simulink model "devCreateSdat"  (R2018b)
settings: Solver=VariableStepDiscrete  StartTime=0  StopTime=1  MaxStep=1  RelTol=1e-3  EnableMultiTasking=on
InitFcn:
  | load('DE_TRY2010_13_averageYear')
libraries: carnot x1, CreateSdat x1
settings Model: Creator=drhf  LastModifiedBy=drhf
settings DataIOCC: SaveFormat=Array  SignalLoggingSaveFormat=ModelDataLogs
settings OptimizationCC: ExpressionDepthLimit=2147483647  LifeSpan=inf
settings DebuggingCC: UnderspecifiedInitializationDetection=Classic  MergeDetectMultiDrivingBlocksExec=none  SolverPrmCheckMsg=warning  FcnCallInpInsideContextMsg=warning  StateNameClashWarn=warning  SFUnexpectedBacktrackingDiag=warning  SFNoUnconditionalDefaultTransitionDiag=warning  SFExecutionAtInitializationDiag=none
settings HardwareCC: ProdBitPerPointer=32  ProdBitPerSizeT=32  ProdBitPerPtrDiffT=32  ProdLargestAtomicFloat=None  ProdIntDivRoundTo=Undefined  ProdEndianess=Unspecified  ProdWordSize=32  ProdHWDeviceType=32-bit Generic
settings ModelReferenceCC: PropagateSignalLabelsOutOfModel=off
settings SFSimCC: SimUseLocalCustomCode=off
settings RTWCC: RTWUseLocalCustomCode=off
settings CodeAppCC: StateflowObjectComments=on
settings GRTTargetCC: TargetLangStandard=C89/C90 (ANSI)  GeneratePreprocessorConditionals=Disable all  CombineOutputUpdateFcns=off  GRTInterface=on
settings ConfigComp: CovMetricSettings=dw  CovHtmlReporting=on  CovSaveCumulativeToWorkspaceVar=on  CovSaveSingleToWorkspaceVar=on  CovExternalEMLEnable=off

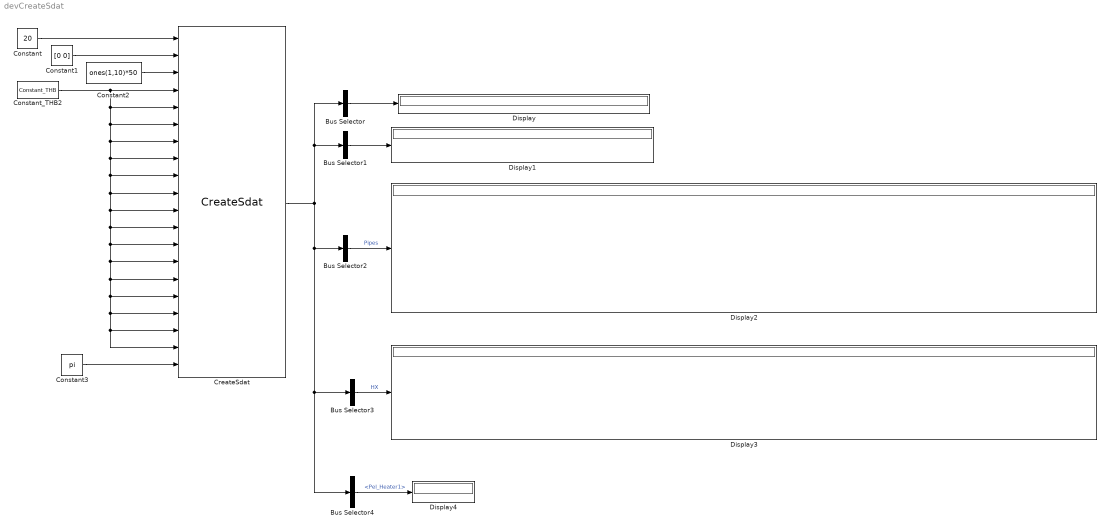
== system devCreateSdat ==
  Bus Selector : BusSelector  OutputSignals=Tamb,energy,volume,storageType  OutputAsBus=on
  Bus Selector1 : BusSelector  OutputSignals=Tnodes  OutputAsBus=on
  Bus Selector2 : BusSelector  OutputSignals=THBin_pipe1,THBout_pipe1,THBin_pipe2,THBout_pipe2,THBin_pipe3,THBout_pipe3,THBin_pipe4,THBout_pipe4,THBin_pipe5,THBout_pipe5  OutputAsBus=on
  Bus Selector3 : BusSelector  OutputSignals=THBin_hx1,THBout_hx1,THBin_hx2,THBout_hx2,THBin_hx3,THBout_hx3  OutputAsBus=on
  Bus Selector4 : BusSelector  OutputSignals=Pel_Heater1
  Constant : Constant  Value=20
  Constant1 : Constant  Value=[0 0]
  Constant2 : Constant  Value=ones(1,10)*50
  Constant3 : Constant  Value=pi
  Constant_THB2 : carnot/Source/Simple/Constant_THB  t=30  mdot=0  p=1e5  mID=No Pressure Drop  fluid=Water  mix=0  mix2=0  mix3=0  dia=0.02  hgt=0
      settings: SourceProductName=Carnot
  CreateSdat : CreateSdat/CreateSdat  volume=0.5  stgtype=1
  Display{,1..4} (5 alike) : Display
  wires:
  CreateSdat/1 -> Bus Selector2/1, Bus Selector3/1, Bus Selector4/1, Bus Selector1/1, Bus Selector/1
  Constant_THB2/1 -> CreateSdat/11, CreateSdat/13, CreateSdat/14, CreateSdat/15, CreateSdat/16, CreateSdat/17, CreateSdat/18, CreateSdat/19, CreateSdat/12, CreateSdat/10, CreateSdat/9, CreateSdat/8, CreateSdat/7, CreateSdat/6, CreateSdat/5, CreateSdat/4
  Constant/1 -> CreateSdat/1
  Constant1/1 -> CreateSdat/2
  Constant2/1 -> CreateSdat/3
  Constant3/1 -> CreateSdat/20
  Bus Selector/1 -> Display/1
  Bus Selector1/1 -> Display1/1
  Bus Selector2/1 -> Display2/1  "Pipes"
  Bus Selector3/1 -> Display3/1  "HX"
  Bus Selector4/1 -> Display4/1  "<Pel_Heater1>"
